simulink model "controller14"  (R2023a)
settings: Solver=FixedStepAuto  StartTime=0.0  StopTime=mdl.rt  RelTol=1e-3
values from neighbouring files (symbols this model uses):
  archived_Eul_XYZ = rst_Eul_XYZ.signals.values    [s4_run.m]    (also in step4_run_v1.m)
  archived_p_raw = rst_p_raw.signals.values    [s4_run.m]    (also in step4_run_v1.m)
  ctr = make_ext_tor_observer(rsim, mdl, ctr)    [s1_setup.m]    (also in setup_controller_with_functions.m = make_controller(); step1_setup.m; step1_setup_v1.m)
  ctr2 = ctr    [s1_setup.m]    (also in step1_setup.m; step1_setup_v1.m)
  lut = gen_lut    [s1_setup.m]    (also in thrust2voltage_lut_20230809.mat = ; thrust2voltage_lut_20230829.mat = )
  mdl = make_model(mdl,rsim)    [s1_setup.m]    (also in setup_controller_with_functions.m = make_model(flight_time); step1_setup.m; step1_setup_v1.m = make_model(flight_time,rsim))
  rbt = make_robot    [s1_setup.m]    (also in setup_controller_with_functions.m = make_robot(); step1_setup.m; step1_setup_v1.m)
  rbt2 = rbt    [s1_setup.m]    (also in step1_setup.m; step1_setup_v1.m)
  rsim = make_robot_simulation()    [setup_controller_with_functions.m]    (also in step1_setup_v1.m = make_simulation(rbt,mdl,rsim))
  som = make_somersault(mdl, rsim)    [s1_setup.m]    (also in step1_setup.m = make_somersault(mdl))
  traj = make_trajectory(ctr, mdl, rsim)    [s1_setup.m]    (also in step1_setup.m)
undefined symbols (not defined in the file or in its folder): DiscIntNeverNeededParam, Standard_Devices, UDP_Protocol
libraries: simulink x27, dspfdesign x7, robotcorelib x6, sldrtlib x4, slrealtimeloglib x1, shared6dof x1, dspsrcs4 x1, uavutilslib x1
(part 3 of 3)

== system controller14/signal generator1/Drive_Signal4/SignalForRamp_binary ==
  note: Should output 1 or -1,
      | so signal ramps UP to 1
      | or DOWN to 0.
  In1 : Inport
  Add : Sum  Inputs=+-
  Compare To Zero : simulink/Logic and Bit Operations/Compare To Zero  relop=>  OutDataTypeStr=uint8  ZeroCross=off
  Constant : Constant
  Data Type Conversion : DataTypeConversion  OutDataTypeStr=double  SaturateOnIntegerOverflow=off  RndMeth=Floor
  Gain : Gain  Gain=2
  Out1 : Outport
  wires:
  In1/1 -> Compare To Zero/1
  Compare To Zero/1 -> Data Type Conversion/1
  Gain/1 -> Add/1
  Constant/1 -> Add/2
  Add/1 -> Out1/1
  Data Type Conversion/1 -> Gain/1

== system controller14/signal generator1/Drive_Signal4/SignalForSin_binary ==
  note: We want this to stay "high" for 1
      | second after the actual "enable"
      | is turned off...
  In1 : Inport
  Compare To Zero : simulink/Logic and Bit Operations/Compare To Zero  relop=>  OutDataTypeStr=uint8  ZeroCross=off
  Data Type Conversion : DataTypeConversion  OutDataTypeStr=double  SaturateOnIntegerOverflow=off  RndMeth=Floor
  Out1 : Outport
  wires:
  In1/1 -> Compare To Zero/1
  Compare To Zero/1 -> Data Type Conversion/1
  Data Type Conversion/1 -> Out1/1

== system controller14/signal generator1/Drive_Signal4/Subsystem ==
  note: positive value pushes the left wing forward
  split cycle mu : Inport
  In2 : Inport  Port=2
  1-mu : Sum  Inputs=+-
  2f : Gain  Gain=2
  2nd harmonic : Trigonometry  OutputSignalType=real
  2pi : Gain  Gain=2*pi
  Abs1 : Abs  SaturateOnIntegerOverflow=off
  Add : Sum
  Constant : Constant
  combined sines : Sum
  deg to rad : Gain  Gain=pi/180
  f : Gain  Gain=-1
  first harmonic : Trigonometry  OutputSignalType=real
  omega*t : DiscreteIntegrator  SampleTime=-1  ICPrevOutput=DiscIntNeverNeededParam  ICPrevScaledInput=DiscIntNeverNeededParam
  phase offset : Constant  Value=0
  signal with gain1 : Product  RndMeth=Zero
  signal with gain2 : Product  RndMeth=Zero
  split cycle signal : Outport
  wires:
  2f/1 -> 2nd harmonic/1
  first harmonic/1 -> signal with gain1/2
  Constant/1 -> 1-mu/1
  split cycle mu/1 -> f/1, Abs1/1
  1-mu/1 -> signal with gain1/1
  2nd harmonic/1 -> signal with gain2/2
  signal with gain1/1 -> combined sines/1
  signal with gain2/1 -> combined sines/2
  combined sines/1 -> split cycle signal/1
  f/1 -> signal with gain2/1
  Abs1/1 -> 1-mu/2
  In2/1 -> 2pi/1
  2pi/1 -> omega*t/1
  omega*t/1 -> Add/2
  Add/1 -> first harmonic/1, 2f/1
  phase offset/1 -> deg to rad/1
  deg to rad/1 -> Add/1

== system controller14/signal generator1/signal generator 1/SignalForRamp_binary ==
  note: Should output 1 or -1,
      | so signal ramps UP to 1
      | or DOWN to 0.
  EnableSignal : Inport
  Add : Sum  Inputs=+-
  Compare To Zero : simulink/Logic and Bit Operations/Compare To Zero  relop=>  OutDataTypeStr=uint8  ZeroCross=off
  Constant : Constant
  Data Type Conversion : DataTypeConversion  OutDataTypeStr=double  SaturateOnIntegerOverflow=off  RndMeth=Floor
  Gain : Gain  Gain=2
  Out1 : Outport
  wires:
  EnableSignal/1 -> Compare To Zero/1
  Compare To Zero/1 -> Data Type Conversion/1
  Gain/1 -> Add/1
  Constant/1 -> Add/2
  Add/1 -> Out1/1
  Data Type Conversion/1 -> Gain/1

== system controller14/signal generator1/signal generator 1/SignalSaturationLimit4 ==
  Max : Inport
  SignalRaw : Inport  Port=2
  MaxOf : MinMax  Function=max  Inputs=2
  MinOf : MinMax  Inputs=2
  ground : Constant
  SignalSatd : Outport
  wires:
  SignalRaw/1 -> MinOf/2
  MinOf/1 -> MaxOf/1
  MaxOf/1 -> SignalSatd/1
  Max/1 -> MinOf/1
  ground/1 -> MaxOf/2

== system controller14/signal generator1/signal generator 1/Subsystem ==
  cos wave : Inport
  new_amplitude : Inport  Port=2
  Delay : Delay  DelayLength=1  InitialCondition=0
  Delay1 : Delay  InitialCondition=[0,0]
  Delay2 : Delay  DelayLength=1  InitialCondition=0
  MATLAB Function : MATLAB Function  TreatAsAtomicUnit=on  SystemSampleTime=mdl.T_high
  output : Outport
  wires:
  cos wave/1 -> Delay1/1, Delay/1, MATLAB Function/1(u1)
  MATLAB Function/1(output) -> output/1, Delay2/1
  Delay/1 -> MATLAB Function/2(u2)
  Delay2/1 -> MATLAB Function/5(old_amplitude)
  Delay1/1 -> MATLAB Function/3(u3)
  new_amplitude/1 -> MATLAB Function/4(new_amplitude)

== system controller14/signal generator1/signal generator 1/get max voltage ==
  note: time constant = 0.002sec
  QuasiEnable : Inport
  max voltage : Inport  Port=2
  Product : Product  RndMeth=Zero
  SIgnalForRamp_binary : Subsystem
  SaturatingRamp : DiscreteIntegrator  gainval=100  SampleTime=-1  LimitOutput=on  UpperSaturationLimit=1  LowerSaturationLimit=0  ICPrevOutput=DiscIntNeverNeededParam  ICPrevScaledInput=DiscIntNeverNeededParam
  max signa; : Outport
  wires:
  Product/1 -> max signa;/1
  max voltage/1 -> Product/2
  QuasiEnable/1 -> SIgnalForRamp_binary/1(In1)
  SIgnalForRamp_binary/1(Out1) -> SaturatingRamp/1
  SaturatingRamp/1 -> Product/1

== system controller14/signal generator1/signal generator 2/SignalForRamp_binary ==
  note: Should output 1 or -1,
      | so signal ramps UP to 1
      | or DOWN to 0.
  EnableSignal : Inport
  Add : Sum  Inputs=+-
  Compare To Zero : simulink/Logic and Bit Operations/Compare To Zero  relop=>  OutDataTypeStr=uint8  ZeroCross=off
  Constant : Constant
  Data Type Conversion : DataTypeConversion  OutDataTypeStr=double  SaturateOnIntegerOverflow=off  RndMeth=Floor
  Gain : Gain  Gain=2
  Out1 : Outport
  wires:
  EnableSignal/1 -> Compare To Zero/1
  Compare To Zero/1 -> Data Type Conversion/1
  Gain/1 -> Add/1
  Constant/1 -> Add/2
  Add/1 -> Out1/1
  Data Type Conversion/1 -> Gain/1

== system controller14/signal generator1/signal generator 2/SignalSaturationLimit4 ==
  Max : Inport
  SignalRaw : Inport  Port=2
  MaxOf : MinMax  Function=max  Inputs=2
  MinOf : MinMax  Inputs=2
  ground : Constant
  SignalSatd : Outport
  wires:
  SignalRaw/1 -> MinOf/2
  MinOf/1 -> MaxOf/1
  MaxOf/1 -> SignalSatd/1
  Max/1 -> MinOf/1
  ground/1 -> MaxOf/2

== system controller14/signal generator1/signal generator 2/Subsystem ==
  cos wave : Inport
  new_amplitude : Inport  Port=2
  Delay : Delay  DelayLength=1  InitialCondition=0
  Delay1 : Delay  InitialCondition=[0,0]
  Delay2 : Delay  DelayLength=1  InitialCondition=0
  MATLAB Function : MATLAB Function  TreatAsAtomicUnit=on  SystemSampleTime=mdl.T_high
  output : Outport
  wires:
  cos wave/1 -> Delay1/1, Delay/1, MATLAB Function/1(u1)
  MATLAB Function/1(output) -> output/1, Delay2/1
  Delay/1 -> MATLAB Function/2(u2)
  Delay2/1 -> MATLAB Function/5(old_amplitude)
  Delay1/1 -> MATLAB Function/3(u3)
  new_amplitude/1 -> MATLAB Function/4(new_amplitude)

== system controller14/signal generator1/signal generator 2/get max voltage ==
  note: time constant = 0.002sec
  QuasiEnable : Inport
  max voltage : Inport  Port=2
  Product : Product  RndMeth=Zero
  SIgnalForRamp_binary : Subsystem
  SaturatingRamp : DiscreteIntegrator  gainval=100  SampleTime=-1  LimitOutput=on  UpperSaturationLimit=1  LowerSaturationLimit=0  ICPrevOutput=DiscIntNeverNeededParam  ICPrevScaledInput=DiscIntNeverNeededParam
  max signa; : Outport
  wires:
  Product/1 -> max signa;/1
  max voltage/1 -> Product/2
  QuasiEnable/1 -> SIgnalForRamp_binary/1(In1)
  SIgnalForRamp_binary/1(Out1) -> SaturatingRamp/1
  SaturatingRamp/1 -> Product/1

== system controller14/signal generator1/signal generator 3/SignalForRamp_binary ==
  note: Should output 1 or -1,
      | so signal ramps UP to 1
      | or DOWN to 0.
  EnableSignal : Inport
  Add : Sum  Inputs=+-
  Compare To Zero : simulink/Logic and Bit Operations/Compare To Zero  relop=>  OutDataTypeStr=uint8  ZeroCross=off
  Constant : Constant
  Data Type Conversion : DataTypeConversion  OutDataTypeStr=double  SaturateOnIntegerOverflow=off  RndMeth=Floor
  Gain : Gain  Gain=2
  Out1 : Outport
  wires:
  EnableSignal/1 -> Compare To Zero/1
  Compare To Zero/1 -> Data Type Conversion/1
  Gain/1 -> Add/1
  Constant/1 -> Add/2
  Add/1 -> Out1/1
  Data Type Conversion/1 -> Gain/1

== system controller14/signal generator1/signal generator 3/SignalSaturationLimit4 ==
  Max : Inport
  SignalRaw : Inport  Port=2
  MaxOf : MinMax  Function=max  Inputs=2
  MinOf : MinMax  Inputs=2
  ground : Constant
  SignalSatd : Outport
  wires:
  SignalRaw/1 -> MinOf/2
  MinOf/1 -> MaxOf/1
  MaxOf/1 -> SignalSatd/1
  Max/1 -> MinOf/1
  ground/1 -> MaxOf/2

== system controller14/signal generator1/signal generator 3/Subsystem ==
  cos wave : Inport
  new_amplitude : Inport  Port=2
  Delay : Delay  DelayLength=1  InitialCondition=0
  Delay1 : Delay  InitialCondition=[0,0]
  Delay2 : Delay  DelayLength=1  InitialCondition=0
  MATLAB Function : MATLAB Function  TreatAsAtomicUnit=on  SystemSampleTime=mdl.T_high
  output : Outport
  wires:
  cos wave/1 -> Delay1/1, Delay/1, MATLAB Function/1(u1)
  MATLAB Function/1(output) -> output/1, Delay2/1
  Delay/1 -> MATLAB Function/2(u2)
  Delay2/1 -> MATLAB Function/5(old_amplitude)
  Delay1/1 -> MATLAB Function/3(u3)
  new_amplitude/1 -> MATLAB Function/4(new_amplitude)

== system controller14/signal generator1/signal generator 3/get max voltage ==
  note: time constant = 0.002sec
  QuasiEnable : Inport
  max voltage : Inport  Port=2
  Product : Product  RndMeth=Zero
  SIgnalForRamp_binary : Subsystem
  SaturatingRamp : DiscreteIntegrator  gainval=100  SampleTime=-1  LimitOutput=on  UpperSaturationLimit=1  LowerSaturationLimit=0  ICPrevOutput=DiscIntNeverNeededParam  ICPrevScaledInput=DiscIntNeverNeededParam
  max signa; : Outport
  wires:
  Product/1 -> max signa;/1
  max voltage/1 -> Product/2
  QuasiEnable/1 -> SIgnalForRamp_binary/1(In1)
  SIgnalForRamp_binary/1(Out1) -> SaturatingRamp/1
  SaturatingRamp/1 -> Product/1

== system controller14/signal generator1/signal generator 4/SignalForRamp_binary ==
  note: Should output 1 or -1,
      | so signal ramps UP to 1
      | or DOWN to 0.
  EnableSignal : Inport
  Add : Sum  Inputs=+-
  Compare To Zero : simulink/Logic and Bit Operations/Compare To Zero  relop=>  OutDataTypeStr=uint8  ZeroCross=off
  Constant : Constant
  Data Type Conversion : DataTypeConversion  OutDataTypeStr=double  SaturateOnIntegerOverflow=off  RndMeth=Floor
  Gain : Gain  Gain=2
  Out1 : Outport
  wires:
  EnableSignal/1 -> Compare To Zero/1
  Compare To Zero/1 -> Data Type Conversion/1
  Gain/1 -> Add/1
  Constant/1 -> Add/2
  Add/1 -> Out1/1
  Data Type Conversion/1 -> Gain/1

== system controller14/signal generator1/signal generator 4/SignalSaturationLimit4 ==
  Max : Inport
  SignalRaw : Inport  Port=2
  MaxOf : MinMax  Function=max  Inputs=2
  MinOf : MinMax  Inputs=2
  ground : Constant
  SignalSatd : Outport
  wires:
  SignalRaw/1 -> MinOf/2
  MinOf/1 -> MaxOf/1
  MaxOf/1 -> SignalSatd/1
  Max/1 -> MinOf/1
  ground/1 -> MaxOf/2

== system controller14/signal generator1/signal generator 4/Subsystem ==
  cos wave : Inport
  new_amplitude : Inport  Port=2
  Delay : Delay  DelayLength=1  InitialCondition=0
  Delay1 : Delay  InitialCondition=[0,0]
  Delay2 : Delay  DelayLength=1  InitialCondition=0
  MATLAB Function : MATLAB Function  TreatAsAtomicUnit=on  SystemSampleTime=mdl.T_high
  output : Outport
  wires:
  cos wave/1 -> Delay1/1, Delay/1, MATLAB Function/1(u1)
  MATLAB Function/1(output) -> output/1, Delay2/1
  Delay/1 -> MATLAB Function/2(u2)
  Delay2/1 -> MATLAB Function/5(old_amplitude)
  Delay1/1 -> MATLAB Function/3(u3)
  new_amplitude/1 -> MATLAB Function/4(new_amplitude)

== system controller14/signal generator1/signal generator 4/get max voltage ==
  note: time constant = 0.002sec
  QuasiEnable : Inport
  max voltage : Inport  Port=2
  Product : Product  RndMeth=Zero
  SIgnalForRamp_binary : Subsystem
  SaturatingRamp : DiscreteIntegrator  gainval=100  SampleTime=-1  LimitOutput=on  UpperSaturationLimit=1  LowerSaturationLimit=0  ICPrevOutput=DiscIntNeverNeededParam  ICPrevScaledInput=DiscIntNeverNeededParam
  max signa; : Outport
  wires:
  Product/1 -> max signa;/1
  max voltage/1 -> Product/2
  QuasiEnable/1 -> SIgnalForRamp_binary/1(In1)
  SIgnalForRamp_binary/1(Out1) -> SaturatingRamp/1
  SaturatingRamp/1 -> Product/1

== system controller14/Control scheme/attitude and thrust controller/Yaw Controller/start ramp ==
  0.8 : Constant  Value=0.01
  2 : Constant  Value=mdl.i_delay
  Add1 : Sum
  Add2 : Sum  Inputs=+-
  Compare To Zero : simulink/Logic and Bit Operations/Compare To Zero  relop=>  OutDataTypeStr=uint8  ZeroCross=off
  Data Type Conversion : DataTypeConversion  SaturateOnIntegerOverflow=off  RndMeth=Floor
  constant : Constant
  counter : DiscreteIntegrator  gainval=1  SampleTime=-1  UpperSaturationLimit=1  LowerSaturationLimit=0  ICPrevOutput=DiscIntNeverNeededParam  ICPrevScaledInput=DiscIntNeverNeededParam
  saturation ramp : DiscreteIntegrator  gainval=5  SampleTime=-1  LimitOutput=on  UpperSaturationLimit=1  LowerSaturationLimit=-1  ICPrevOutput=DiscIntNeverNeededParam  ICPrevScaledInput=DiscIntNeverNeededParam
  Out1 : Outport
  wires:
  constant/1 -> counter/1
  2/1 -> Add1/1
  0.8/1 -> Add1/2
  counter/1 -> Add2/1
  Add1/1 -> Add2/2
  Add2/1 -> Compare To Zero/1
  Compare To Zero/1 -> Data Type Conversion/1
  saturation ramp/1 -> Out1/1
  Data Type Conversion/1 -> saturation ramp/1

== system controller14/Control scheme/observer/Rotaion/filtered derivative ==
  In1 : Inport
  att_s : Gain  Gain=mdl.f1
  filtered derivative : simulink/Discrete/Transfer Fcn Lead or Lag  PoleZ=mdl.zf1  ZeroZ=1  ICPrevOutput=0.0  ICPrevInput=0.0  DoSatur=off
  low pass3 : DiscreteTransferFcn  Numerator=mdl.vlp.n  Denominator=mdl.vlp.d
  Out1 : Outport
  wires:
  filtered derivative/1 -> low pass3/1
  att_s/1 -> filtered derivative/1
  In1/1 -> att_s/1
  low pass3/1 -> Out1/1

== system controller14/Control scheme/observer/lateral observer/saturation ==
  In1 : Inport
  MinMax2 : MinMax  Inputs=2
  MinMax3 : MinMax  Function=max  Inputs=2
  lw1 : Constant  Value=-mdl.fd_lim
  up1 : Constant  Value=mdl.fd_lim
  Out1 : Outport
  wires:
  In1/1 -> MinMax2/2
  up1/1 -> MinMax2/1
  lw1/1 -> MinMax3/1
  MinMax2/1 -> MinMax3/2
  MinMax3/1 -> Out1/1

== system controller14/signal generator1/signal generator 1/get max voltage/SIgnalForRamp_binary ==
  note: Should output 1 or -1,
      | so signal ramps UP to 1
      | or DOWN to 0.
  In1 : Inport
  Add : Sum  Inputs=+-
  Compare To Zero : simulink/Logic and Bit Operations/Compare To Zero  relop=>  OutDataTypeStr=uint8  ZeroCross=off
  Constant : Constant
  Data Type Conversion : DataTypeConversion  OutDataTypeStr=double  SaturateOnIntegerOverflow=off  RndMeth=Floor
  Gain : Gain  Gain=2
  Out1 : Outport
  wires:
  In1/1 -> Compare To Zero/1
  Compare To Zero/1 -> Data Type Conversion/1
  Gain/1 -> Add/1
  Constant/1 -> Add/2
  Add/1 -> Out1/1
  Data Type Conversion/1 -> Gain/1

== system controller14/signal generator1/signal generator 2/get max voltage/SIgnalForRamp_binary ==
  note: Should output 1 or -1,
      | so signal ramps UP to 1
      | or DOWN to 0.
  In1 : Inport
  Add : Sum  Inputs=+-
  Compare To Zero : simulink/Logic and Bit Operations/Compare To Zero  relop=>  OutDataTypeStr=uint8  ZeroCross=off
  Constant : Constant
  Data Type Conversion : DataTypeConversion  OutDataTypeStr=double  SaturateOnIntegerOverflow=off  RndMeth=Floor
  Gain : Gain  Gain=2
  Out1 : Outport
  wires:
  In1/1 -> Compare To Zero/1
  Compare To Zero/1 -> Data Type Conversion/1
  Gain/1 -> Add/1
  Constant/1 -> Add/2
  Add/1 -> Out1/1
  Data Type Conversion/1 -> Gain/1

== system controller14/signal generator1/signal generator 3/get max voltage/SIgnalForRamp_binary ==
  note: Should output 1 or -1,
      | so signal ramps UP to 1
      | or DOWN to 0.
  In1 : Inport
  Add : Sum  Inputs=+-
  Compare To Zero : simulink/Logic and Bit Operations/Compare To Zero  relop=>  OutDataTypeStr=uint8  ZeroCross=off
  Constant : Constant
  Data Type Conversion : DataTypeConversion  OutDataTypeStr=double  SaturateOnIntegerOverflow=off  RndMeth=Floor
  Gain : Gain  Gain=2
  Out1 : Outport
  wires:
  In1/1 -> Compare To Zero/1
  Compare To Zero/1 -> Data Type Conversion/1
  Gain/1 -> Add/1
  Constant/1 -> Add/2
  Add/1 -> Out1/1
  Data Type Conversion/1 -> Gain/1

== system controller14/signal generator1/signal generator 4/get max voltage/SIgnalForRamp_binary ==
  note: Should output 1 or -1,
      | so signal ramps UP to 1
      | or DOWN to 0.
  In1 : Inport
  Add : Sum  Inputs=+-
  Compare To Zero : simulink/Logic and Bit Operations/Compare To Zero  relop=>  OutDataTypeStr=uint8  ZeroCross=off
  Constant : Constant
  Data Type Conversion : DataTypeConversion  OutDataTypeStr=double  SaturateOnIntegerOverflow=off  RndMeth=Floor
  Gain : Gain  Gain=2
  Out1 : Outport
  wires:
  In1/1 -> Compare To Zero/1
  Compare To Zero/1 -> Data Type Conversion/1
  Gain/1 -> Add/1
  Constant/1 -> Add/2
  Add/1 -> Out1/1
  Data Type Conversion/1 -> Gain/1

== matlab function controller14/Subsystem/MATLAB Function ==
  data: t input; enable output; mdl parameter
function enable = fcn(t, mdl)

if t > mdl.i_delay && t < (mdl.i_delay + mdl.flight_time)
    enable = 1;
else
    enable = 0;
end

end

== matlab function controller14/Archived data for rerun/MATLAB Function1 ==
  data: t input; y output; archived_data_ready parameter
function y = fcn(t,archived_data_ready)

t = floor(t);
y = archived_data_ready(t,1);

end

== matlab function controller14/Archived data for rerun/MATLAB Function2 ==
  data: t input; y output; archived_p_raw parameter; archived_Eul_XYZ parameter
function y = fcn(t,archived_p_raw,archived_Eul_XYZ)

y = zeros(6,1);

t = floor(t);
y(1:3,1) = archived_p_raw(t,1:3)';
y(4:6,1) = archived_Eul_XYZ(t,1:3)';

end

== matlab function controller14/Control scheme/attitude and thrust controller/Subsystem/MATLAB Function ==
  data: time input; en_int output; ctr parameter; mdl parameter
function en_int = fcn(time, ctr, mdl)

    if ctr.takeoff.en
        wait_time = ctr.takeoff.time;
    else
        wait_time = 0;
    end
    
    if time > (mdl.i_delay + wait_time) && ctr.integral.en
        en_int = 1;
    else 
        en_int = 0;
    end

end

== matlab function controller14/back mapping from sat volt to torque-thrust/power_distribution_1 ==
  data: motor_thrust input; torque_thrust output; rbt parameter
function torque_thrust  = fcn(motor_thrust, rbt)

% motor_thrust is in mgf
torque_x_mgfm = (- motor_thrust(1) + motor_thrust(2) ...
                 + motor_thrust(3) - motor_thrust(4)) * rbt.lt; % (mgf*m)
torque_y_mgfm = (- motor_thrust(1) - motor_thrust(2) ...
                 + motor_thrust(3) + motor_thrust(4)) * rbt.ld; % (mgf*m)
thrust_mgf    = (+ motor_thrust(1) + motor_thrust(2) ...
                 + motor_thrust(3) + motor_thrust(4)); % (mgf)        

% convert mgf to N (mgf*m & N*m)
torque = [torque_x_mgfm; torque_y_mgfm; 0] * 9.81e-6; %(N*m)
thrust = thrust_mgf * 9.81e-6; % (N)

torque_thrust = [torque; thrust];

% ==== original code ====
% r = torque(1) / roll_arm;
% p = torque(2) / pitch_arm; % (mgf) = (mgf*m) / (m)
% 
% att = [
%     - r - p;
%     + r - p;
%     + r + p;
%     - r + p]; % (mgf)
% 
% min_t = min(att);
% 
% if (thrust < - min_t)
%     thrust = - min_t; 
% end
%     
% m1 = thrust + att(1); % (mgf)
% m2 = thrust + att(2); % (mgf)
% m3 = thrust + att(3); % (mgf)
% m4 = thrust + att(4); % (mgf)
% 
% 
% motors_thrust = [m1; m2; m3; m4]; % (mgf)
% 
% return;
end

== matlab function controller14/motor thrust mapping ==
  data: torque input; motors_thrust output; total_thrust input; rbt parameter
function motors_thrust = fcn(torque, total_thrust, rbt)

% torque in mgf*m
% total_thrust in mgf

% thrust of each unit
thrust = total_thrust/4;

% get force from body x/y axis torque  (consider moment arm)
r = torque(1) / rbt.lt / 4; % force on each unit (mgf)
p = torque(2) / rbt.ld / 4; % force on each unit (mgf)

% map force to each unit
att = [
    - r - p;
    + r - p;
    + r + p;
    - r + p];

% prioritize attitude over thrust
min_att  = min(att);
if (thrust < - min_att)
    thrust = - min_att; 
end

% map thrust and torque to each unit 
m1 = thrust + att(1);
m2 = thrust + att(2);
m3 = thrust + att(3);
m4 = thrust + att(4);

% create vector
motors_thrust = [m1; m2; m3; m4];

return;
end

== matlab function controller14/Control scheme/adaptive setpoint rd ==
  data: r input; rd output size=3; rd_d output size=3; rd_dd output size=3; rd_ddd output size=3; rd_dddd output size=3; init_r_out output size=3; time input; init_r_in input; id_in input; ctr2 parameter; mdl parameter; id_out output size=1; traj parameter
function [rd,rd_d,rd_dd,rd_ddd,rd_dddd,init_r_out, id_out] = fcn(r, time, init_r_in, id_in, ctr2, mdl, traj)

    % this function defines desired setpoint for the model-based controller

    persistent id init_r
    
    if isempty(id) 
        id = 1;
    else
        id = id +1;
    end

    if isempty(init_r) 
        init_r = zeros(3,1);
    end
    
    % initialize output variables
    rd      = zeros(3,1); % postion
    rd_d    = zeros(3,1); % velocity
    rd_dd   = zeros(3,1); % acceleration
    rd_ddd  = zeros(3,1); % jerk
    rd_dddd = zeros(3,1); % snap

    % get initial position of the robot
    if time < mdl.i_delay
        init_r_out = r(:);
        init_r = r(:);
    else
        init_r_out = init_r_in(:);
    end

    % update id
    id_in   = floor(id_in);
    id_out  = id_in + 1;
    
    if ~traj.en
    
        % == no trajectory following (just takeoff and landing) ==
        rd = [init_r(1) + ctr2.setpoint.x;...
              init_r(2) + ctr2.setpoint.y;...
              init_r(3) + ctr2.setpoint.z];

        init_height = init_r(3) + 0.003;
        
        % befor takeoff
        if time <= mdl.i_delay+0.03
            rd   = [init_r(1) + ctr2.setpoint.x;...
                    init_r(2) + ctr2.setpoint.y;...
                    init_height];
        end
        
        % takeoff
        if ctr2.takeoff.en
            if time > mdl.i_delay+0.03 && time < (mdl.i_delay+0.03+ctr2.takeoff.time)
                
                % rd_z (desired position)
                rd_z = init_height + (((init_r(3) + ctr2.setpoint.z-init_height)/ctr2.takeoff.time)*(time-mdl.i_delay-0.03));
                if rd_z > init_r(3) + ctr2.setpoint.z
                    rd_z = init_r(3) + ctr2.setpoint.z;
                end
                rd(3)  = rd_z;
                
                % rd_d_z (desired velocity)
                rd_d_z = ((init_r(3) + ctr2.setpoint.z-init_height)/ctr2.takeoff.time);
                rd_d   = [rd_d(1); rd_d(2); rd_d_z];
                
            end
        end
        
        % planned landing 
        if ctr2.landing.en
            if time > ((mdl.i_delay+mdl.flight_time)-ctr2.landing.time)
                
                % rd_z (desired position)
                rd_z = init_r(3) + ctr2.setpoint.z-(((init_r(3) + ctr2.setpoint.z-init_height)/ctr2.landing.time)*(time-(mdl.i_delay+mdl.flight_time)+ctr2.landing.time));
                if rd_z < init_height
                    rd_z = init_height;
                end
                rd(3)  =  rd_z;
                
                % rd_d_z (desired velocity)
                rd_d_z = (init_height-ctr2.setpoint.z-init_r(3))/ctr2.landing.time;
                rd_d   = [rd_d(1); rd_d(2); rd_d_z];
                
            end
        end

    else

        % == use pre-defined trajectory ==
       
        % use predefined trajectory
        if traj.en
            rd      = init_r + traj.rd(1:3,id);
            rd_d    = traj.rd_d(1:3,id);
            rd_dd   = traj.rd_dd(1:3,id);
            rd_ddd  = traj.rd_ddd(1:3,id);
            rd_dddd = traj.rd_dddd(1:3,id);
        end

    end



end

% somersault
% if som.en
%     if time > som.t_start + som.t_rise + som.t_acc + som.t_dcc + som.t_rec
%         % % afterwards 
%         %dt = som.t_start + som.t_rise + som.t_acc + som.t_dcc + som.t_rec - time;
%         %rd = rd + dt*(r-rd);
%     elseif time > som.t_start + som.t_rise + som.t_acc + som.t_dcc
%         % recovery
%         dt = som.t_start + som.t_rise + som.t_acc + som.t_dcc + som.t_rec - time;
%         rd = rd + (dt/som.t_rec)*(r-rd);
%         rd_d = rd_d + 0.5*(dt/som.t_rec)*(r_d-rd_d);
%         rd(1) = min(max(rd(1),-0.25),0.25); % 25 cm envelope
%         rd(2) = min(max(rd(2),-0.25),0.25); % 25 cm envelope
%         rd(3) = max(rd(3),0.02); % min altitude setpoint.
%     end
% end

== matlab function controller14/Safety check/safety check system/MATLAB Function ==
  data: keep_flying input; en_in input; en_out output size=1; cum_in input; cum_out output size=1; ctr parameter; mdl parameter
function [en_out, cum_out] = fcn(keep_flying, en_in, cum_in, ctr, mdl)

if keep_flying == 0
    cum_out = cum_in + mdl.T;
else
    cum_out = 0;
end

if cum_out > ctr.safety.T || en_in == 0
    en_out = 0;
else 
    en_out = 1;
end

end

== matlab function controller14/Safety check/safety check system/envelope check ==
  data: x input; en output; y input; z input; ctr parameter
function en  = fcn(x,y,z, ctr)

if abs(x)>ctr.safety.enableZone.xmax || abs(y)>ctr.safety.enableZone.ymax || abs(z)>ctr.safety.enableZone.zmax
    en = 0;
else
    en = 1;
end

end

== matlab function controller14/Safety check/safety check system/voltage check ==
  data: voltage input; en output; ctr parameter
function en  = fcn(voltage, ctr)

    if sum(voltage>ctr.safety.volt) > 0
        en = 0;
    else
        en = 1;
    end

end

== matlab function controller14/Control scheme/attitude and thrust controller/Controller ==
  data: r input; torque_x output size=1; r_dot input; r_dotdot input; R input; Omega input; rd input; rd_d input; rd_dd input; rd_ddd input; rd_dddd input; ext_torq input; int_tf input; time input; ctr parameter; rbt parameter; torque_y output size=1; torque_z output size=1; F output; torque_gyro output; mdl parameter; att_e output; alt_e output; traj parameter; som parameter; state output; debug1 output; debug2 output; debug3 output; debug4 output
function [torque_x, torque_y, torque_z, F, torque_gyro, att_e, alt_e, state, debug1, debug2,debug3, debug4] = fcn(r, r_dot, r_dotdot, R, Omega, rd,rd_d,rd_dd,rd_ddd,rd_dddd, ext_torq, int_tf, time, ctr, rbt, mdl, traj, som)
    
% ==================================
% ==== preliminary =================
% ==================================
    persistent id som_state
    
    if isempty(id) 
        id = 1;
    else
        id = id +1;
    end

    if isempty(som_state) 
        som_state = 0;
    end

    % get compact notation
    R1     = R(:,1);
    R2     = R(:,2);
    R3     = R(:,3);
    wx     = Omega(1);
    wy     = Omega(2);
    wz     = Omega(3);
    w      = Omega(:);
    Dr     = r-rd;
    Dr_dot = r_dot-rd_d;
    J      = diag([rbt.ixx, rbt.iyy, rbt.izz]);
    eulZXY = rotm2eul(R,'ZYX');
    eulx   = eulZXY(3);


% ==================================
% ==== somersault state ============
% ==================================
    if som.en

        % som_state == 0 is nominal hovering controller
        
        % get into translational acceleration
        if som_state == 0 && time >= som.t.acc % && r_dot(3) < som.threshold.z_dot.acc
            som_state = 1;
        
        % get into flip acceleration
        elseif som_state == 1 && r_dot(3) >= som.threshold.z_dot.acc
            som_state = 2;

        % get into flip deceleration
        elseif som_state == 2 && eulx >= som.threshold.down.eulx && R(3,3) <= som.threshold.down.R33
            som_state = 3;

        % get into translational deceleration
        elseif som_state == 3 && R(3,3) >= som.threshold.up.R33
            som_state = 4;

        % get into nominal hovering controller
        elseif som_state == 4 && r_dot(3) > som.threshold.z_dot.dec
            som_state = 5;
        end
    end


% ==================================
% ==== lateral controller ==========
% ==================================

    % get thrust correction  
    acc_net_b = 0;

    if ctr.atmg.en
        acc_net_b = traj.thrust_b(id); % thrust for aggresive traj
    end

    if som.en
        if som_state == 1 
            acc_net_b = som.thrust.acc * rbt.m; % accelerate at the predetermined value
        elseif som_state == 4 
            acc_net_b = som.thrust.dec * rbt.m; % accelerate at the predetermined value
        end
    end

    % set gain
    if som.en
        if som_state == 3
            ctr.torque_obs.factor.y = 0;
        elseif som_state == 4
            ctr.gain.at3 = ctr.gain.at3 * som.gain.fact.at3;
            ctr.gain.at2 = ctr.gain.at2 * som.gain.fact.at2;
            ctr.gain.at1 = ctr.gain.at1 * som.gain.fact.at1;
            ctr.gain.at0 = ctr.gain.at0 * som.gain.fact.at0;
            ctr.torque_obs.factor.x = 0;
            ctr.torque_obs.factor.y = 0;
        end
    end
    
    % % get desired angular accelaration
    des_wx_dot = (- dot(R2,rd_dddd)  ...
                  - ctr.gain.at3*( (mdl.g+max(-0.1,0))*wx+dot(R2,rd_ddd) )  ...
                  - ctr.gain.at2*( dot(R2,mdl.g*[0;0;1]+rd_dd) )  ...
                  + ctr.gain.at1*( dot(R2,Dr_dot) )  ...
                  + ctr.gain.at0*( dot(R2,Dr) )  ...
                  + int_tf(1)) ...
                  /((mdl.g+max(-0.5,acc_net_b*ctr.gain.atmg.factor.x))); % 

    des_wy_dot = (+ dot(R1,rd_dddd)  ...
                  - ctr.gain.at3*( (mdl.g+max(-0.1,0))*wy-dot(R1,rd_ddd) )  ...
                  - ctr.gain.at2*( dot(R1,-mdl.g*[0;0;1]-rd_dd) )  ...
                  - ctr.gain.at1*( dot(R1,Dr_dot) )  ...
                  - ctr.gain.at0*( dot(R1,Dr) ) ...
                  + int_tf(2)) ...
                  / ((mdl.g+max(-0.5,acc_net_b*ctr.gain.atmg.factor.x))); % + ...

    % gyropscopic effect (might be noisy)
    torque_gyro = J*[des_wx_dot; des_wy_dot; 0] + cross(w,J*w);

    % just moment of inertia
    torque = J*[des_wx_dot; des_wy_dot; 0];

    % get torque
    torque_x = torque(1) - ext_torq(1)*ctr.torque_obs.factor.x + ctr.torque_offset.x;
    torque_y = torque(2) - ext_torq(2)*ctr.torque_obs.factor.y + ctr.torque_offset.y;
    torque_z = 0; % no yaw control

    % original Pakpong controller
    % torque_x = -dot(R2,rd_dddd)  ...
    %     - ctr.gain.at3*( (mdl.g+max(-0.1,acc_net_b))*wx+dot(R2,rd_ddd) )  ...
    %     - ctr.gain.at2*( dot(R2,mdl.g*[0;0;1]+rd_dd) )  ...
    %     + ctr.gain.at1*( dot(R2,Dr_dot) )  ...
    %     + ctr.gain.at0*( dot(R2,Dr) )  ...
    %     + int_tf(1); %  ...
    %     %- ctr.gain.atfd * dot(R2,traj.rd(:,id));
    % 
    % torque_x = torque_x*rbt.ixx/(mdl.g+max(-0.5,acc_net_b*ctr.gain.atmg.factor.x)) - ext_torq(1)*ctr.torque_obs.factor.x + ctr.torque_offset.x;
    % 
    % torque_y = dot(R1,rd_dddd)  ...
    %     - ctr.gain.at3*( (mdl.g+max(-0.1,acc_net_b))*wy-dot(R1,rd_ddd) )  ...
    %     - ctr.gain.at2*( dot(R1,-mdl.g*[0;0;1]-rd_dd) )  ...
    %     - ctr.gain.at1*( dot(R1,Dr_dot) )  ...
    %     - ctr.gain.at0*( dot(R1,Dr) ) ...
    %     + int_tf(2);  %...
    %     %+ ctr.gain.atfd * dot(R1,traj.rd(:,id));
    % 
    % 
    % torque_y = torque_y*rbt.iyy/(mdl.g+max(-0.5,acc_net_b*ctr.gain.atmg.factor.y)) - ext_torq(2)*ctr.torque_obs.factor.y + ctr.torque_offset.y;
    % % +rd_dd(3)
    % torque_z = 0;           % no yaw control


% ==================================
% ==== altitude controller =========
% ==================================
    
    % linear feedforward (for the tether weight)
    ffwd = mdl.g * max(0,rd(3)*ctr.gain.alfd);
    
    % desired net acceleration for the 2nd-order system (not taking r_dotdot)
    a_net = rd_dd(3) - ctr.gain.al1*( r_dot(3)-rd_d(3) ) - ctr.gain.al0*( r(3)-rd(3) );
    
    % gravity + net acceleration + integral term + feedforward
    a_w = mdl.g + a_net + int_tf(4) + ffwd + ctr.thrust_offset; % world frame

    % world to body frame
    a_b = a_w/R(3,3);

    % saturation
    a = max(min(a_b, mdl.g+4), mdl.g-4.0); % during hovering.

    % convert accelearation to Newton
    F = a*rbt.m;


% ==================================
% ==== intergral error =============
% ==================================

    % attitude error
    att_e = [dot(R2,Dr);-dot(R1,Dr);0];

    % altitude error
    alt_e = -( r(3)-rd(3) )/R(3,3);


% ==================================
% ==== somersault torque/thrsut ====
% ==================================

    if som.en
        
        % translational acceleration
        if som_state == 1
            F = som.thrust.acc * rbt.m;

        % flip acceleration
        elseif som_state == 2
            torque_x = som.tor_x.acc;
            torque_y = 0;
            F = 0;

        % flip deceleration
        elseif som_state == 3
            % if eulx < (-pi*1/2)
            %     torque_x = som.tor_x.dec;
            % else
            %     torque_x = (0-eulx)*3.5478e-06*49 + (0-wx)*7.8840e-07*1;
            % end
            if eulx > 2
                eulx = eulx - (2*pi);
            end
            torque_x = + (0-eulx) * som.tor_x.gain.dec.p ...
                       + (0-wx) * som.tor_x.gain.dec.d;
            % torque_x = som.tor_x.dec;
            F = 0;

        % translational deceleration
        elseif som_state == 4
            F = som.thrust.dec * rbt.m;

        end

    end
    
% torque_gyro = ones(3,1);
state = som_state;
debug1 = ctr.gain.at1;
debug2 = R(3,3);
debug3 = eulx;
debug4 = eulZXY;
 end

== matlab function controller14/State filters/Subsystem5/Rotation Matrix ==
  data: euler_angles input; R output
function R = fcn(euler_angles)
%#codegen

eu_x = euler_angles(1);
eu_y = euler_angles(2);
eu_z = euler_angles(3);

R = [cos(eu_y)*cos(eu_z); -cos(eu_y)*sin(eu_z); sin(eu_y); ...
    cos(eu_x)*sin(eu_z)+sin(eu_x)*sin(eu_y)*cos(eu_z); cos(eu_x)*cos(eu_z)-sin(eu_x)*sin(eu_y)*sin(eu_z); -sin(eu_x)*cos(eu_y); ...
    sin(eu_x)*sin(eu_z)-cos(eu_x)*sin(eu_y)*cos(eu_z); sin(eu_x)*cos(eu_z)+cos(eu_x)*sin(eu_y)*sin(eu_z); cos(eu_x)*cos(eu_y)];


end

% R is 9x1

% Pakpong was using "XYZ" convention, which seems to be the same as Vicon

== matlab function controller14/Control scheme/attitude and thrust controller/External Torque Observer ==
  data: ext_torque_hat output; omega input; omega_hat output; torque_x input; torque_y input; ext_torque_hat input; omega_hat input; time input; ctr2 parameter; rbt2 parameter; mdl parameter
function [ext_torque_hat, omega_hat] = fcn(omega, torque_x, torque_y, ext_torque_hat, omega_hat, time, ctr2, rbt2, mdl)
    
omega_hat           = omega_hat(:);
ext_torque_hat      = ext_torque_hat(:);
J                   = diag([rbt2.ixx, rbt2.iyy, rbt2.izz]);
omega_cross_J_omega = cross(omega, J*omega);
x_hat_curr          = diag(ctr2.torque_obs.state_scaling)*[omega_hat(:); ext_torque_hat(:)];

% til = 20;

% if rbt2.til == 0
u              = diag(ctr2.torque_obs.input_scaling)*[torque_x - omega_cross_J_omega(1); torque_y - omega_cross_J_omega(2)];
y              = diag(ctr2.torque_obs.meas_scaling)*omega(1:2); 
x_hat_pred     = ctr2.torque_obs.A*x_hat_curr + ctr2.torque_obs.B(:, 1:2)*u; 
x_hat_next     = diag(ctr2.torque_obs.out_scaling)*(x_hat_pred + ctr2.torque_obs.L*(y - ctr2.torque_obs.C*x_hat_pred));
omega_hat      = x_hat_next(1:2,1);
ext_torque_hat = x_hat_next(3:4,1);
if time < mdl.i_delay
    omega_hat      = zeros(2,1);
    ext_torque_hat = zeros(2,1);
end
% else
%     u              = diag(ctr2.torque_obs.input_scaling)*[torque_x - omega_cross_J_omega(1); torque_y - omega_cross_J_omega(2); torque_z - omega_cross_J_omega(3)];
%     y              = diag(ctr2.torque_obs.meas_scaling)*omega(1:3); 
%     x_hat_pred     = ctr2.torque_obs.A*x_hat_curr + ctr2.torque_obs.B(:, 1:3)*u; 
%     x_hat_next     = diag(ctr2.torque_obs.out_scaling)*(x_hat_pred + ctr2.torque_obs.L*(y - ctr2.torque_obs.C*x_hat_pred));
%     omega_hat      = x_hat_next(1:3,1);
%     ext_torque_hat = x_hat_next(4:6,1);
%     if time < mdl.i_delay
%         omega_hat      = zeros(3,1);
%         ext_torque_hat = zeros(3,1);
%     end
% end



end

== matlab function controller14/Control scheme/attitude and thrust controller/Thrust Controller ==
  data: r input; F output size=1; r_dot input; r_dotdot input; R input; Omega input; rd input; rd_d input; rd_dd input; rd_ddd input; rd_dddd input; int_tf input; mdl parameter; ctr parameter; alt_e output size=1; rbt parameter
function [F, alt_e]  = fcn(r, r_dot, r_dotdot, R, Omega, rd,rd_d,rd_dd,rd_ddd,rd_dddd, int_tf, mdl, ctr, rbt)

    % initialize
    R33 = R(9); % body to world
    
    % linear feedforward (for the tether weight)
    ffwd = mdl.g * max(0,rd(3)*ctr.gain.alfd);
    
    % desired net acceleration for the 2nd-order system (not taking r_dotdot)
    a_net = rd_dd(3) - ctr.gain.al1*( r_dot(3)-rd_d(3) ) - ctr.gain.al0*( r(3)-rd(3) );
    
    % gravity + net acceleration + integral term + feedforward
    a_w = mdl.g + a_net + int_tf(4) + ffwd + ctr.thrust_offset;

    % world to body frame
    a_b = a_w/R33;

    % saturation
    a = max(min(a_b, mdl.g+4), mdl.g-4.0); % during hovering.

    % convert accelearation to Newton
    F = a*rbt.m;
    
    % get intergral error
    alt_e = -( r(3)-rd(3) )/R33;

    % somersault
    if som.en
        
        % accelerate at the predetermined value
        if time > som.t1 && <= som.t2
            F = som.acc * rbt.m; 

        % no thrust during flipping
        elseif time > som.t2 && time <= som.t3
            F = 0;
            

        end

        

    end

end

== matlab function controller14/Control scheme/attitude and thrust controller/Yaw Controller/MATLAB Function ==
  data: torq_ext input; torq_z input; torq_z output; ctr2 parameter; rbt2 parameter
function torq_z = fcn(torq_ext,torq_z,ctr2, rbt2)

if rbt2.til > 0
    if ctr2.yaw.dy.en == 0
%         torq_z = torq_z - torq_ext(3) * ctr2.torque_obs.factor.z;
    end
else
    torq_z = torq_z;
end

end

== matlab function controller14/Control scheme/attitude and thrust controller/Yaw Controller/desired yaw ==
  data: t input; id input; rd_yaw output; ctr2 parameter; index output; mdl parameter
function [rd_yaw, index] = fcn(t,id,ctr2,mdl)

if ctr2.yaw.dy.en
    
    if id > 1
        t_cum = sum(ctr2.yaw.dy.duration(1:id-1))+sum(ctr2.yaw.dy.trans(1:id-1));
    else
        t_cum = 0;
    end

    if t > mdl.i_delay + t_cum && t <= mdl.i_delay + t_cum + ctr2.yaw.dy.duration(id)
        rd_yaw = ctr2.yaw.dy.angle(id);
    elseif t > mdl.i_delay + t_cum + ctr2.yaw.dy.duration(id) && t < mdl.i_delay + t_cum + ctr2.yaw.dy.duration(id) + ctr2.yaw.dy.trans(id)
        rd_yaw = ctr2.yaw.dy.angle(id) + (ctr2.yaw.dy.angle(id+1)-ctr2.yaw.dy.angle(id))/ctr2.yaw.dy.trans(id)*(t-mdl.i_delay-t_cum-ctr2.yaw.dy.duration(id));
    elseif t >= mdl.i_delay + t_cum + ctr2.yaw.dy.duration(id) + ctr2.yaw.dy.trans(id)
        rd_yaw = ctr2.yaw.dy.angle(id+1);
        id = id + 1;
    else
        rd_yaw = 0;
    end

else
    
    rd_yaw = ctr2.setpoint.yaw;
    
end

index = id;
    
end

== matlab function controller14/Control scheme/observer/Rotaion/Rotation Matrix ==
  data: euler_angles input; R output
function R = fcn(euler_angles)
%#codegen

eu_x = euler_angles(1);
eu_y = euler_angles(2);
eu_z = euler_angles(3);

R = [cos(eu_y)*cos(eu_z); -cos(eu_y)*sin(eu_z); sin(eu_y); ...
    cos(eu_x)*sin(eu_z)+sin(eu_x)*sin(eu_y)*cos(eu_z); cos(eu_x)*cos(eu_z)-sin(eu_x)*sin(eu_y)*sin(eu_z); -sin(eu_x)*cos(eu_y); ...
    sin(eu_x)*sin(eu_z)-cos(eu_x)*sin(eu_y)*cos(eu_z); sin(eu_x)*cos(eu_z)+cos(eu_x)*sin(eu_y)*sin(eu_z); cos(eu_x)*cos(eu_y)];
% R is 1x9

== matlab function controller14/Control scheme/observer/Rotaion/Rotation Matrix1 ==
  data: R input; Rdot input; w output
function w  = fcn(R,Rdot)
%#codegen
w = zeros(3,1);
w(1) = R(3)*Rdot(2) + R(6)*Rdot(5) + R(9)*Rdot(8);
w(2) = R(1)*Rdot(3) + R(4)*Rdot(6) + R(7)*Rdot(9);
w(3) = R(2)*Rdot(1) + R(5)*Rdot(4) + R(8)*Rdot(7);

== matlab function controller14/Control scheme/saturation ==
  data: x_roll input; X_roll output size=1; y_pitch input; z_yaw input; Y_pitch output size=1; Z_yaw output size=1; F input; Force output size=1; ctr2 parameter
function [X_roll, Y_pitch, Z_yaw, Force] = fcn(x_roll, y_pitch, z_yaw, F, ctr2)


    X_roll = max(min(x_roll, ctr2.lim.taux), -ctr2.lim.taux);
    
    Y_pitch = max(min(y_pitch, ctr2.lim.tauy), -ctr2.lim.tauy);
    
    Z_yaw = max(min(z_yaw, ctr2.lim.tauz), -ctr2.lim.tauz);
    
    Force = F;

end

% F is already checked for saturation

  
% Thrust management
% thrust is not controlled during the flipping maneuver (the output here will be overridden in the mapping).

== matlab function controller14/State filters/Subsystem5/Rotation Matrix2 ==
  data: R input; Rdot input; w output
function w  = fcn(R,Rdot)
%#codegen
w = zeros(3,1);
w(1) = R(3)*Rdot(2) + R(6)*Rdot(5) + R(9)*Rdot(8);
w(2) = R(1)*Rdot(3) + R(4)*Rdot(6) + R(7)*Rdot(9);
w(3) = R(2)*Rdot(1) + R(5)*Rdot(4) + R(8)*Rdot(7);

% w = R^T * dot(R)

end

== matlab function controller14/State filters/Subsystem5/Rotation Matrix3 ==
  data: R input; Rdot input; w output
function w  = fcn(R,Rdot)
%#codegen
w = zeros(3,1);
w(1) = R(3)*Rdot(2) + R(6)*Rdot(5) + R(9)*Rdot(8);
w(2) = R(1)*Rdot(3) + R(4)*Rdot(6) + R(7)*Rdot(9);
w(3) = R(2)*Rdot(1) + R(5)*Rdot(4) + R(8)*Rdot(7);

% w = R^T * dot(R)

end

== matlab function controller14/signal generator1/signal generator 4/Subsystem/MATLAB Function ==
  data: u1 input; output output; u2 input; u3 input; new_amplitude input; old_amplitude input
function output  = fcn(u1, u2, u3, new_amplitude, old_amplitude)

if u2 < u1 && u2 < u3
    output = new_amplitude;
else
    output = old_amplitude;
end

    
end

== matlab function controller14/signal generator1/signal generator 3/Subsystem/MATLAB Function ==
  data: u1 input; output output; u2 input; u3 input; new_amplitude input; old_amplitude input
function output  = fcn(u1, u2, u3, new_amplitude, old_amplitude)

if u2 < u1 && u2 < u3
    output = new_amplitude;
else
    output = old_amplitude;
end

    
end

== matlab function controller14/signal generator1/signal generator 2/Subsystem/MATLAB Function ==
  data: u1 input; output output; u2 input; u3 input; new_amplitude input; old_amplitude input
function output  = fcn(u1, u2, u3, new_amplitude, old_amplitude)

if u2 < u1 && u2 < u3
    output = new_amplitude;
else
    output = old_amplitude;
end

    
end

== matlab function controller14/signal generator1/signal generator 1/Subsystem/MATLAB Function ==
  data: u1 input; output output; u2 input; u3 input; new_amplitude input; old_amplitude input
function output  = fcn(u1, u2, u3, new_amplitude, old_amplitude)

if u2 < u1 && u2 < u3
    output = new_amplitude;
else
    output = old_amplitude;
end

    
end
